simulink model "Comparacion_ANN"  (R2021a)
settings: Solver=VariableStepAuto  StartTime=0.0  StopTime=60  RelTol=1e-4
values from neighbouring files (symbols this model uses):
  selector = i    [Simulation.m]
undefined symbols (not defined in the file or in its folder): sigbuilder_block
libraries: spsDiodeLib x5, spsPVArrayLib x5, deeplib x4, simulink x4, spsCurrentMeasurementLib x1, spsControlledVoltageSourceLib x1, spsVoltageMeasurementLib x1, spspowerguiLib x1
settings Model: Creator=Guillermo  LastModifiedBy=Guillermo

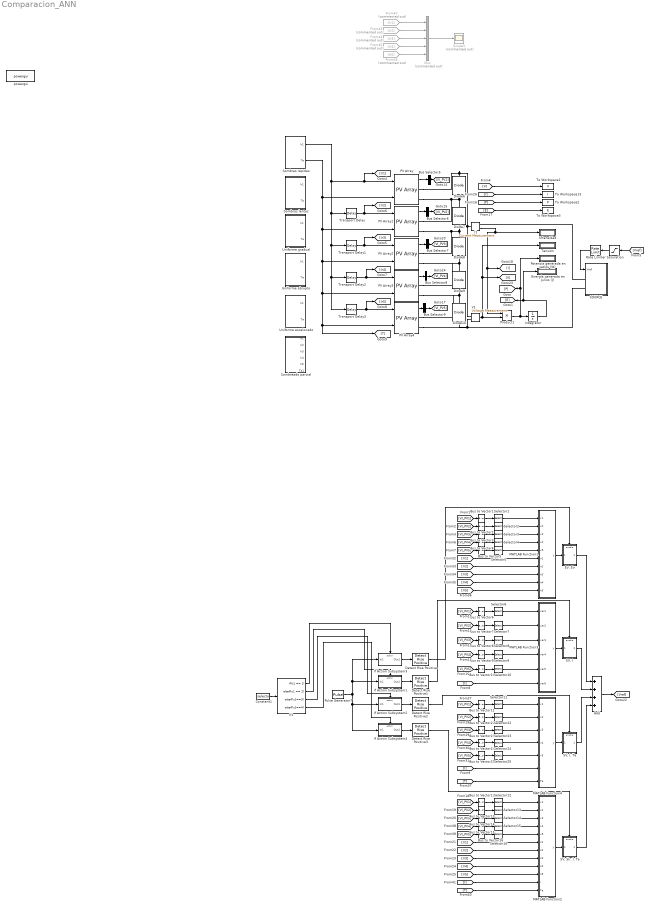
== system Comparacion_ANN ==
  "5V, 5Ir" : Subsystem
  "5V, 5Ir, I, Ta" : Subsystem
  "5V, I" : Subsystem
  "5V, I, Ta" : Subsystem
  Add : Sum  Inputs=++++
  Bus Selector{5..9} (5 alike) : BusSelector  OutputSignals=V_PV,I_PV  OutputAsBus=on
  Bus to Vector{1..16,22..25} (20 alike) : BusToVector
  Constant1 : Constant  Value=selector
  Detect Rise Positive{,1..3} (4 alike) : simulink/Logic and Bit Operations/Detect Rise Positive  vinit=0  OutDataTypeStr=boolean
  Diode{6..10} (5 alike) : spsDiodeLib/Diode  Ron=0.001  Lon=0  Vf=0.7  IC=0  UseSnubber=off  Rs=1e5*inf  Cs=inf  Measurements=off
  "Energía generada en Julios (J) " : Display
  From42 : From  Commented=on  GotoTag=Ir1
  From43 : From  Commented=on  GotoTag=Ir2
  From44 : From  Commented=on  GotoTag=Ir3
  From45 : From  Commented=on  GotoTag=Ir4
  From46 : From  Commented=on  GotoTag=Ir5
  I1 : spsCurrentMeasurementLib/Current Measurement  PhasorSimulation=off  OutputType=Complex  PSBequivalent=0
  If Action Subsystem1 : Subsystem  TreatAsAtomicUnit=on
  If Action Subsystem2 : Subsystem  TreatAsAtomicUnit=on
  If Action Subsystem3 : Subsystem  TreatAsAtomicUnit=on
  If Action Subsystem4 : Subsystem  TreatAsAtomicUnit=on
  If1 : If  IfExpression=u1 == 1  ElseIfExpressions=u1 == 2, u1==3, u1==4  ShowElse=off
  Integrator : Integrator
  Intensidad : Display
  MATLAB Function1 : MATLAB Function  TreatAsAtomicUnit=on
  MATLAB Function2 : MATLAB Function  TreatAsAtomicUnit=on
  MATLAB Function3 : MATLAB Function  TreatAsAtomicUnit=on
  MATLAB Function4 : MATLAB Function  TreatAsAtomicUnit=on
  Mux : Mux  Commented=on  Inputs=5
  PV Array{,1..4} (5 alike) : spsPVArrayLib/PV Array  Npar=1  Nser=1  PlotType=array @ 1000 W/m2 & specified temperatures  S_vec="[ 1000  500  100 ]"  Temp_C_vec="[ 45 25  ]"  ModuleName=SunPower SPR-305E-WHT-D  PlotWhenSelected=off  Pm=305.226  Ncell=96  Voc=64.2  Isc=5.96  Vm=54.7  Im=5.58  beta_Voc_pc=-0.2727  alpha_Isc_pc=0.061745  beta_Voc=-0.17507  alpha_Isc=0.00368  IL=5.9657  I0=6.3076e-12  nI=0.94489  Rsh=393.2054  Rs=0.37428  RobustModel=off  RobustCellTemperature=313.3991  BAL=on  Tc=1e-3  Tfilter=5e-5
  "Potencia generada en vatios (W) " : Display
  Product1 : Product
  Pulse Generator7 : DiscretePulseGenerator  PulseType=Time based  Period=1e-3  PulseWidth=20
      settings: AttributesFormatString=Period: %<period>\nDuty cycle: %<pulsewidth>%
  Rate Limiter : RateLimiter  RisingSlewLimit=100000  FallingSlewLimit=-100000  SampleTimeMode=inherited  InitialCondition=150
  SOURCE : Subsystem
  Saturation : Saturate  UpperLimit=290  LowerLimit=40
  Scope3 : Scope  Commented=on
  Selector{1..16,22..25} (20 alike) : Selector  InputPortWidth=2  IndexOptions=Index vector (dialog)  Indices=[1]  OutputSizes=1
  Sombras lentas : Subsystem  Tag=STV Subsys  LoadFcn=sigbuilder_block('load');  StartFcn=sigbuilder_block('start');  StopFcn=sigbuilder_block('stop');  ClipboardFcn=sigbuilder_block('clipboard');  mask(Sigbuilder block){tuvar=[0:10]}
      mask help: Simulink:masks:SigbuilderBlock_MD
      mask init:
      | if ~strcmp(get_param(bdroot(gcbh),'SimulationStatus'),'stopped') tuvar = sigbuilder_block('maskInit'); end
      settings: CopyFcn=sigbuilder_block('copy');  DeleteFcn=sigbuilder_block('delete');  ModelCloseFcn=sigbuilder_block('modelClose');  PreSaveFcn=sigbuilder_block('preSave');  PauseFcn=sigbuilder_block('pause');  ContinueFcn=sigbuilder_block('continue');  NameChangeFcn=sigbuilder_block('namechange');  OpenFcn=sigbuilder_block('open',[6 30 1908 951.75 ]);  CloseFcn=sigbuilder_block('close');
      mask Display: plot(0, 0, 100, 100,[2, 2, 32, 32, 2], [68, 8, 8, 68, 68],[32, 2], [38, 38], [32, 19, 2],[53, 60, 44], [32, 17, 17, 2],[16, 16, 31, 31]);txt = getActiveGroup(gcbh);text(2, 100, txt,'verticalAlignment', 'top');
  Sombras rápidas : Subsystem  Tag=STV Subsys  LoadFcn=sigbuilder_block('load');  StartFcn=sigbuilder_block('start');  StopFcn=sigbuilder_block('stop');  ClipboardFcn=sigbuilder_block('clipboard');  mask(Sigbuilder block){tuvar=[0:10]}
      mask help: Simulink:masks:SigbuilderBlock_MD
      mask init:
      | if ~strcmp(get_param(bdroot(gcbh),'SimulationStatus'),'stopped') tuvar = sigbuilder_block('maskInit'); end
      settings: CopyFcn=sigbuilder_block('copy');  DeleteFcn=sigbuilder_block('delete');  ModelCloseFcn=sigbuilder_block('modelClose');  PreSaveFcn=sigbuilder_block('preSave');  PauseFcn=sigbuilder_block('pause');  ContinueFcn=sigbuilder_block('continue');  NameChangeFcn=sigbuilder_block('namechange');  OpenFcn=sigbuilder_block('open',[6 30 1908 951.75 ]);  CloseFcn=sigbuilder_block('close');
      mask Display: plot(0, 0, 100, 100,[2, 2, 32, 32, 2], [68, 8, 8, 68, 68],[32, 2], [38, 38], [32, 19, 2],[53, 60, 44], [32, 17, 17, 2],[16, 16, 31, 31]);txt = getActiveGroup(gcbh);text(2, 100, txt,'verticalAlignment', 'top');
  Sombreado parcial : Subsystem  Tag=STV Subsys  LoadFcn=sigbuilder_block('load');  StartFcn=sigbuilder_block('start');  StopFcn=sigbuilder_block('stop');  ClipboardFcn=sigbuilder_block('clipboard');  mask(Sigbuilder block){tuvar=[0:10]}
      mask help: Simulink:masks:SigbuilderBlock_MD
      mask init:
      | if ~strcmp(get_param(bdroot(gcbh),'SimulationStatus'),'stopped') tuvar = sigbuilder_block('maskInit'); end
      settings: CopyFcn=sigbuilder_block('copy');  DeleteFcn=sigbuilder_block('delete');  ModelCloseFcn=sigbuilder_block('modelClose');  PreSaveFcn=sigbuilder_block('preSave');  PauseFcn=sigbuilder_block('pause');  ContinueFcn=sigbuilder_block('continue');  NameChangeFcn=sigbuilder_block('namechange');  OpenFcn=sigbuilder_block('open',[6 30 1908 951.75 ]);  CloseFcn=sigbuilder_block('close');
      mask Display: plot(0, 0, 100, 100,[2, 2, 32, 32, 2], [68, 8, 8, 68, 68],[32, 2], [38, 38], [32, 19, 2],[53, 60, 44], [32, 17, 17, 2],[16, 16, 31, 31]);txt = getActiveGroup(gcbh);text(2, 100, txt,'verticalAlignment', 'top');
  Tensión : Display
  To Workspace1 : ToWorkspace  VariableName=V  SampleTime=1e-3
  To Workspace13 : ToWorkspace  VariableName=I  SampleTime=1e-3
  To Workspace2 : ToWorkspace  VariableName=P  SampleTime=1e-3
  To Workspace3 : ToWorkspace  VariableName=E  SampleTime=1e-3
  Transport Delay : TransportDelay  DelayTime=0.1  InitialOutput=1000
  Transport Delay1 : TransportDelay  DelayTime=0.2  InitialOutput=1000
  Transport Delay2 : TransportDelay  DelayTime=0.3  InitialOutput=1000
  Transport Delay3 : TransportDelay  DelayTime=0.4  InitialOutput=1000
  Uniforme abrupto : Subsystem  Tag=STV Subsys  LoadFcn=sigbuilder_block('load');  StartFcn=sigbuilder_block('start');  StopFcn=sigbuilder_block('stop');  ClipboardFcn=sigbuilder_block('clipboard');  mask(Sigbuilder block){tuvar=[0:10]}
      mask help: Simulink:masks:SigbuilderBlock_MD
      mask init:
      | if ~strcmp(get_param(bdroot(gcbh),'SimulationStatus'),'stopped') tuvar = sigbuilder_block('maskInit'); end
      settings: CopyFcn=sigbuilder_block('copy');  DeleteFcn=sigbuilder_block('delete');  ModelCloseFcn=sigbuilder_block('modelClose');  PreSaveFcn=sigbuilder_block('preSave');  PauseFcn=sigbuilder_block('pause');  ContinueFcn=sigbuilder_block('continue');  NameChangeFcn=sigbuilder_block('namechange');  OpenFcn=sigbuilder_block('open',[6 30 1908 951.75 ]);  CloseFcn=sigbuilder_block('close');
      mask Display: plot(0, 0, 100, 100,[2, 2, 32, 32, 2], [68, 8, 8, 68, 68],[32, 2], [38, 38], [32, 19, 2],[53, 60, 44], [32, 17, 17, 2],[16, 16, 31, 31]);txt = getActiveGroup(gcbh);text(2, 100, txt,'verticalAlignment', 'top');
  Uniforme escalonado : Subsystem  Tag=STV Subsys  LoadFcn=sigbuilder_block('load');  StartFcn=sigbuilder_block('start');  StopFcn=sigbuilder_block('stop');  ClipboardFcn=sigbuilder_block('clipboard');  mask(Sigbuilder block){tuvar=[0:10]}
      mask help: Simulink:masks:SigbuilderBlock_MD
      mask init:
      | if ~strcmp(get_param(bdroot(gcbh),'SimulationStatus'),'stopped') tuvar = sigbuilder_block('maskInit'); end
      settings: CopyFcn=sigbuilder_block('copy');  DeleteFcn=sigbuilder_block('delete');  ModelCloseFcn=sigbuilder_block('modelClose');  PreSaveFcn=sigbuilder_block('preSave');  PauseFcn=sigbuilder_block('pause');  ContinueFcn=sigbuilder_block('continue');  NameChangeFcn=sigbuilder_block('namechange');  OpenFcn=sigbuilder_block('open',[6 30 1908 951.75 ]);  CloseFcn=sigbuilder_block('close');
      mask Display: plot(0, 0, 100, 100,[2, 2, 32, 32, 2], [68, 8, 8, 68, 68],[32, 2], [38, 38], [32, 19, 2],[53, 60, 44], [32, 17, 17, 2],[16, 16, 31, 31]);txt = getActiveGroup(gcbh);text(2, 100, txt,'verticalAlignment', 'top');
  Uniforme gradual : Subsystem  Tag=STV Subsys  LoadFcn=sigbuilder_block('load');  StartFcn=sigbuilder_block('start');  StopFcn=sigbuilder_block('stop');  ClipboardFcn=sigbuilder_block('clipboard');  mask(Sigbuilder block){tuvar=[0:10]}
      mask help: Simulink:masks:SigbuilderBlock_MD
      mask init:
      | if ~strcmp(get_param(bdroot(gcbh),'SimulationStatus'),'stopped') tuvar = sigbuilder_block('maskInit'); end
      settings: CopyFcn=sigbuilder_block('copy');  DeleteFcn=sigbuilder_block('delete');  ModelCloseFcn=sigbuilder_block('modelClose');  PreSaveFcn=sigbuilder_block('preSave');  PauseFcn=sigbuilder_block('pause');  ContinueFcn=sigbuilder_block('continue');  NameChangeFcn=sigbuilder_block('namechange');  OpenFcn=sigbuilder_block('open',[6 30 1908 951.75 ]);  CloseFcn=sigbuilder_block('close');
      mask Display: plot(0, 0, 100, 100,[2, 2, 32, 32, 2], [68, 8, 8, 68, 68],[32, 2], [38, 38], [32, 19, 2],[53, 60, 44], [32, 17, 17, 2],[16, 16, 31, 31]);txt = getActiveGroup(gcbh);text(2, 100, txt,'verticalAlignment', 'top');
  V1 : spsVoltageMeasurementLib/Voltage Measurement  PhasorSimulation=off  OutputType=Complex  PSBequivalent=0
  powergui : spspowerguiLib/powergui  Priority=1  SimulationMode=Continuous  SampleTime=1e-7  frequency=60  Iterations=50  frequencyindice=0  Pbase=100e6  ErrMax=1e-4  UnitsV=kV  UnitsW=MW  buscounter=0  FunctionMessages=off  echomessages=off  EnableUseOfTLC=off  CurrentSourceSwitches=off  DisableSnubberDevices=on  DisableRonSwitches=off  DisableVfSwitches=off  DisplayEquations=off  AutomaticDiscreteSolvers=off  SolverType=Tustin/Backward Euler (TBE)  Interpol=off  ExternalGateDelay=off  methode=off  Ts=0  x0status=blocks  SPID=off  SwTol=0  HookPort=off  NonlinearTolerance=1e-4  nMaxIteration=100  ContinueOnMaxIteration=off  RestoreLinks=warning  ResistiveCurrentMeasurement=off  Frange=[0:2:500]  Ylog=off  Xlog=on  ShowGrid=off  save=off  variable=ZData  structure=0  ZoomFFT=on  StartTime=0.0  cycles=1  DisplayStyle=1  fundamental=60  FreqAxis=off  MaxFrequency=1000  frequencyindicesteady=1  RmsSteady=1  display=off
  wires:
  Bus Selector9/1 -> [VI_PV5]
  Bus Selector7/1 -> [VI_PV3]
  [I] -> MATLAB Function3/6(var6)
  Bus Selector5/1 -> [VI_PV1]
  [T] -> MATLAB Function4/7(Ta)
  [I] -> MATLAB Function4/6(i)
  V1/1 -> Tensión/1, [V], Product1/2
  PV Array2/1 -> Bus Selector7/1
  [I] -> To Workspace13/1
  Bus Selector8/1 -> [VI_PV4]
  [V] -> To Workspace1/1
  PV Array3/1 -> Bus Selector8/1
  Bus Selector6/1 -> [VI_PV2]
  PV Array/1 -> Bus Selector5/1
  PV Array1/1 -> Bus Selector6/1
  I1/1 -> Product1/1, [I], Intensidad/1
  PV Array4/1 -> Bus Selector9/1
  Integrator/1 -> "Energía generada en Julios (J) "/1, [E]
  Product1/1 -> [P], "Potencia generada en vatios (W) "/1, Integrator/1
  Bus to Vector4/1 -> Selector4/1
  Bus to Vector2/1 -> Selector2/1
  [VI_PV1] -> Bus to Vector1/1
  Bus to Vector3/1 -> Selector3/1
  [VI_PV3] -> Bus to Vector3/1
  Bus to Vector1/1 -> Selector1/1
  Bus to Vector5/1 -> Selector5/1
  Selector1/1 -> MATLAB Function1/1(v1)
  Selector5/1 -> MATLAB Function1/5(v5)
  Selector4/1 -> MATLAB Function1/4(v4)
  [VI_PV4] -> Bus to Vector4/1
  [VI_PV5] -> Bus to Vector5/1
  Selector3/1 -> MATLAB Function1/3(v3)
  [VI_PV2] -> Bus to Vector2/1
  Selector2/1 -> MATLAB Function1/2(v2)
  Bus to Vector9/1 -> Selector9/1
  Bus to Vector7/1 -> Selector7/1
  [VI_PV1] -> Bus to Vector6/1
  Bus to Vector8/1 -> Selector8/1
  [VI_PV3] -> Bus to Vector8/1
  Bus to Vector6/1 -> Selector6/1
  Bus to Vector10/1 -> Selector10/1
  Selector6/1 -> MATLAB Function3/1(var1)
  Selector10/1 -> MATLAB Function3/5(var5)
  Selector9/1 -> MATLAB Function3/4(var4)
  [VI_PV4] -> Bus to Vector9/1
  [VI_PV5] -> Bus to Vector10/1
  Selector8/1 -> MATLAB Function3/3(var3)
  [VI_PV2] -> Bus to Vector7/1
  Selector7/1 -> MATLAB Function3/2(var2)
  Bus to Vector24/1 -> Selector24/1
  Bus to Vector22/1 -> Selector22/1
  [VI_PV1] -> Bus to Vector11/1
  Bus to Vector23/1 -> Selector23/1
  [VI_PV3] -> Bus to Vector23/1
  Bus to Vector11/1 -> Selector11/1
  Bus to Vector25/1 -> Selector25/1
  Selector11/1 -> MATLAB Function4/1(v1)
  Selector25/1 -> MATLAB Function4/5(v5)
  Selector24/1 -> MATLAB Function4/4(v4)
  [VI_PV4] -> Bus to Vector24/1
  [VI_PV5] -> Bus to Vector25/1
  Selector23/1 -> MATLAB Function4/3(v3)
  [VI_PV2] -> Bus to Vector22/1
  Selector22/1 -> MATLAB Function4/2(v2)
  [Ir5] -> MATLAB Function1/10(ir5)
  [Ir4] -> MATLAB Function1/9(ir4)
  [Ir3] -> MATLAB Function1/8(ir3)
  [Ir2] -> MATLAB Function1/7(ir2)
  [Ir1] -> MATLAB Function1/6(ir1)
  [P] -> To Workspace2/1
  [E] -> To Workspace3/1
  "5V, 5Ir"/1(Out1) -> Add/1
  MATLAB Function1/1(y) -> "5V, 5Ir"/1(In1)
  MATLAB Function3/1(y) -> "5V, I"/1(In1)
  "5V, I"/1(Out1) -> Add/2
  MATLAB Function4/1(y) -> "5V, I, Ta"/1(In1)
  "5V, I, Ta"/1(Out1) -> Add/3
  "5V, 5Ir, I, Ta"/1(Out1) -> Add/4
  MATLAB Function2/1(y) -> "5V, 5Ir, I, Ta"/1(In1)
  Selector15/1 -> MATLAB Function2/4(v4)
  [Ir1] -> MATLAB Function2/6(ir1)
  [Ir2] -> MATLAB Function2/7(ir2)
  [Ir3] -> MATLAB Function2/8(ir3)
  Bus to Vector16/1 -> Selector16/1
  [Ir4] -> MATLAB Function2/9(ir4)
  [Ir5] -> MATLAB Function2/10(ir5)
  Bus to Vector13/1 -> Selector13/1
  Bus to Vector12/1 -> Selector12/1
  Bus to Vector15/1 -> Selector15/1
  Selector14/1 -> MATLAB Function2/3(v3)
  [VI_PV5] -> Bus to Vector16/1
  Selector16/1 -> MATLAB Function2/5(v5)
  [VI_PV2] -> Bus to Vector13/1
  [VI_PV1] -> Bus to Vector12/1
  Bus to Vector14/1 -> Selector14/1
  Selector12/1 -> MATLAB Function2/1(v1)
  Selector13/1 -> MATLAB Function2/2(v2)
  [VI_PV3] -> Bus to Vector14/1
  [VI_PV4] -> Bus to Vector15/1
  [T] -> MATLAB Function2/12(Ta)
  [I] -> MATLAB Function2/11(i)
  From45/1 -> Mux/4
  From46/1 -> Mux/5
  From42/1 -> Mux/1
  From43/1 -> Mux/2
  From44/1 -> Mux/3
  Mux/1 -> Scope3/1
  Saturation/1 -> Rate Limiter/1
  Constant1/1 -> If1/1
  If Action Subsystem1/1(Out1) -> Detect Rise Positive1/1
  If Action Subsystem2/1(Out1) -> Detect Rise Positive2/1
  If Action Subsystem4/1(Out1) -> Detect Rise Positive3/1
  If1/2 -> If Action Subsystem1/Action
  Pulse Generator7/1 -> If Action Subsystem3/1(In1), If Action Subsystem1/1(In1), If Action Subsystem4/1(In1), If Action Subsystem2/1(In1)
  If1/1 -> If Action Subsystem3/Action
  If1/3 -> If Action Subsystem2/Action
  If1/4 -> If Action Subsystem4/Action
  Detect Rise Positive1/1 -> "5V, I"/Enable
  Detect Rise Positive/1 -> "5V, 5Ir"/Enable
  Detect Rise Positive2/1 -> "5V, I, Ta"/Enable
  Detect Rise Positive3/1 -> "5V, 5Ir, I, Ta"/Enable
  Add/1 -> [Vref]
  Transport Delay/1 -> [Ir2], PV Array1/1
  Transport Delay1/1 -> PV Array2/1, [Ir3]
  Transport Delay2/1 -> [Ir4], PV Array3/1
  Transport Delay3/1 -> [Ir5], PV Array4/1
  Sombras rápidas/1(Ir1) -> Transport Delay3/1, Transport Delay2/1, Transport Delay1/1, Transport Delay/1, [Ir1], PV Array/1
  Sombras rápidas/2(Ta) -> PV Array/2, PV Array1/2, PV Array2/2, PV Array3/2, PV Array4/2, [T]
  [Vref] -> Saturation/1
  Rate Limiter/1 -> SOURCE/1(Vref)
  If Action Subsystem3/1(Out1) -> Detect Rise Positive/1
  connections:
  PV Array4/RConn1 -- PV Array3/RConn2 -- Diode10/RConn1 -- Diode9/LConn1
  Diode7/RConn1 -- Diode6/LConn1 -- PV Array1/RConn1 -- PV Array/RConn2
  SOURCE/LConn2 -- PV Array4/RConn2 -- Diode10/LConn1 -- V1/LConn2
  Diode8/RConn1 -- Diode7/LConn1 -- PV Array2/RConn1 -- PV Array1/RConn2
  Diode6/RConn1 -- I1/LConn1 -- V1/LConn1 -- PV Array/RConn1
  PV Array3/RConn1 -- PV Array2/RConn2 -- Diode9/RConn1 -- Diode8/LConn1
  SOURCE/LConn1 -- I1/RConn1

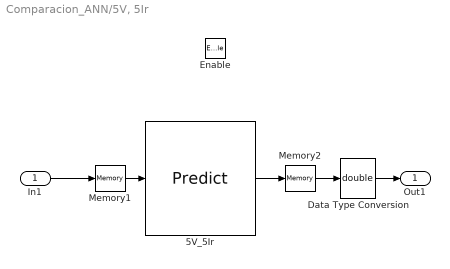
== system Comparacion_ANN/5V, 5Ir ==
  In1 : Inport
  Enable : EnablePort
  5V_5Ir : deeplib/Predict  Network=Network from MAT-file  NetworkFunction=squeezenet  NetworkFilePath=D:\Guillermo\Documentos\Universidad\TFG_E\MATLAB_FINAL\Comparacion_modelos_ANN\modelos_matlab\3_layers\5V_5Ir.mat  MiniBatchSize=256  InputDataFormats={ '', '' }  Predictions=on  Activations={}  ForceInterpretedSim=off  EnableDLNetwork=off
      settings: SourceProductBaseCode=NN
  Data Type Conversion : DataTypeConversion  OutDataTypeStr=double
  Memory1 : Memory
  Memory2 : Memory
  Out1 : Outport
  wires:
  Memory1/1 -> 5V_5Ir/1
  5V_5Ir/1 -> Memory2/1
  Memory2/1 -> Data Type Conversion/1
  In1/1 -> Memory1/1
  Data Type Conversion/1 -> Out1/1

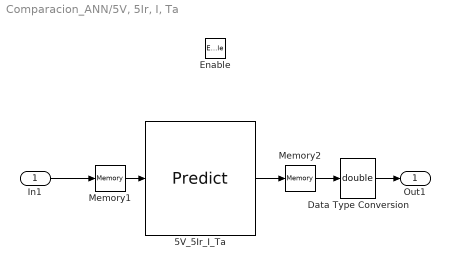
== system Comparacion_ANN/5V, 5Ir, I, Ta ==
  In1 : Inport
  Enable : EnablePort
  5V_5Ir_I_Ta : deeplib/Predict  Network=Network from MAT-file  NetworkFunction=squeezenet  NetworkFilePath=D:\Guillermo\Documentos\Universidad\TFG_E\MATLAB_FINAL\Comparacion_modelos_ANN\modelos_matlab\3_layers\5V_5Ir_I_Ta.mat  MiniBatchSize=256  InputDataFormats={ '', '' }  Predictions=on  Activations={}  ForceInterpretedSim=off  EnableDLNetwork=off
      settings: SourceProductBaseCode=NN
  Data Type Conversion : DataTypeConversion  OutDataTypeStr=double
  Memory1 : Memory
  Memory2 : Memory
  Out1 : Outport
  wires:
  Memory1/1 -> 5V_5Ir_I_Ta/1
  5V_5Ir_I_Ta/1 -> Memory2/1
  Memory2/1 -> Data Type Conversion/1
  In1/1 -> Memory1/1
  Data Type Conversion/1 -> Out1/1

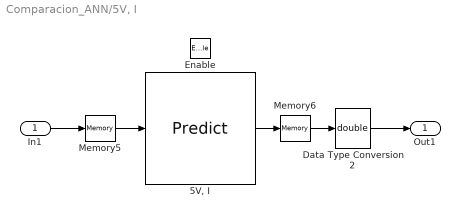
== system Comparacion_ANN/5V, I ==
  In1 : Inport
  Enable : EnablePort
  "5V, I" : deeplib/Predict  Network=Network from MAT-file  NetworkFunction=squeezenet  NetworkFilePath=D:\Guillermo\Documentos\Universidad\TFG_E\MATLAB_FINAL\Comparacion_modelos_ANN\modelos_matlab\3_layers\5V_I.mat  MiniBatchSize=256  InputDataFormats={ '', '' }  Predictions=on  Activations={}  ForceInterpretedSim=off  EnableDLNetwork=off
      settings: SourceProductBaseCode=NN
  Data Type Conversion2 : DataTypeConversion  OutDataTypeStr=double
  Memory5 : Memory
  Memory6 : Memory
  Out1 : Outport
  wires:
  Memory5/1 -> "5V, I"/1
  Memory6/1 -> Data Type Conversion2/1
  Data Type Conversion2/1 -> Out1/1
  "5V, I"/1 -> Memory6/1
  In1/1 -> Memory5/1

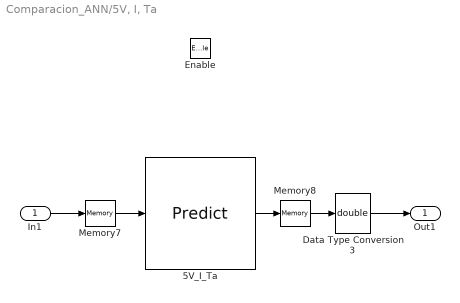
== system Comparacion_ANN/5V, I, Ta ==
  In1 : Inport
  Enable : EnablePort
  5V_I_Ta : deeplib/Predict  Network=Network from MAT-file  NetworkFunction=squeezenet  NetworkFilePath=D:\Guillermo\Documentos\Universidad\TFG_E\MATLAB_FINAL\Comparacion_modelos_ANN\modelos_matlab\3_layers\5V_I_Ta.mat  MiniBatchSize=256  InputDataFormats={ '', '' }  Predictions=on  Activations={}  ForceInterpretedSim=off  EnableDLNetwork=off
      settings: SourceProductBaseCode=NN
  Data Type Conversion3 : DataTypeConversion  OutDataTypeStr=double
  Memory7 : Memory
  Memory8 : Memory
  Out1 : Outport
  wires:
  Data Type Conversion3/1 -> Out1/1
  Memory7/1 -> 5V_I_Ta/1
  5V_I_Ta/1 -> Memory8/1
  Memory8/1 -> Data Type Conversion3/1
  In1/1 -> Memory7/1

== system Comparacion_ANN/If Action Subsystem1 ==
  In1 : Inport
  Action Port : ActionPort  InitializeStates=reset  ActionPortLabel=elseif(u1 == 2)
  Out1 : Outport
  wires:
  In1/1 -> Out1/1

== system Comparacion_ANN/If Action Subsystem2 ==
  In1 : Inport
  Action Port : ActionPort  InitializeStates=reset  ActionPortLabel=elseif( u1==3)
  Out1 : Outport
  wires:
  In1/1 -> Out1/1

== system Comparacion_ANN/If Action Subsystem3 ==
  In1 : Inport
  Action Port : ActionPort  InitializeStates=reset  ActionPortLabel=if(u1 == 1)
  Out1 : Outport
  wires:
  In1/1 -> Out1/1

== system Comparacion_ANN/If Action Subsystem4 ==
  In1 : Inport
  Action Port : ActionPort  InitializeStates=reset  ActionPortLabel=elseif( u1==4)
  Out1 : Outport
  wires:
  In1/1 -> Out1/1

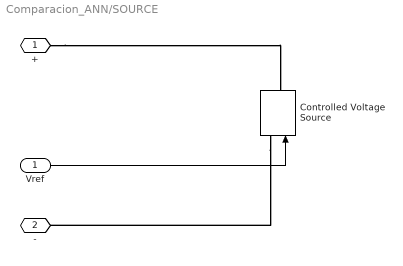
== system Comparacion_ANN/SOURCE ==
  Vref : Inport
  Controlled Voltage Source : spsControlledVoltageSourceLib/Controlled Voltage Source  Initialize=on  Source_Type=AC  Amplitude=0  Phase=0  Frequency=0  Measurements=None
  + : PMIOPort  Side=Left
  - : PMIOPort  Port=2  Side=Left
  wires:
  Vref/1 -> Controlled Voltage Source/1
  connections:
  Controlled Voltage Source/LConn1 -- -/RConn1
  +/RConn1 -- Controlled Voltage Source/RConn1

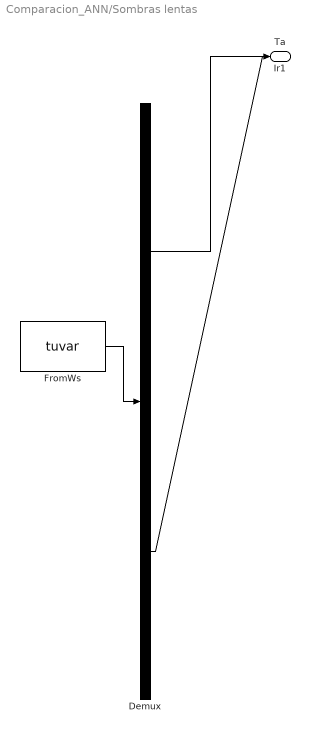
== system Comparacion_ANN/Sombras lentas ==
  Demux : Demux  Tag=STV Demux  Outputs=2
      settings: DisplayOption=none
  FromWs : FromWorkspace  Tag=STV FromWs  VariableName=tuvar
      SigBuilderData=|
      | common.afterFinalStr = 'Extrapolate'
      | common.sampleTime = 0
      | dataSet.timeRange = [0 60]
      | dataSet.name = 'Group 1'
      | sbobj.Groups.Name = 'Group 1'
      | sbobj.Groups.Signals(1).Name = 'Ir1'
      | sbobj.Groups.Signals(1).XData = [0 1 1.4 7 7.25 16.5 16.75 25.25 25.75 34.75 35 37 37.25 45 45.25 48 48.25 50 50.25 57 57.25 60]
      | sbobj.Groups.Signals(1).YData = [910 500 295 295 910 910 295 295 910 910 295 295 910 910 295 295 910 910 295 295 910 910]
      | sbobj.Groups.Signals(2).Name = 'Ta'
      | sbobj.Groups.Signals(2).XData = [0 60]
      | sbobj.Groups.Signals(2).YData = [22.6 22.6]
      | sbobj.Groups.TimeRange = [0 60]
  Ir1 : Outport  Tag=STV Outport
  Ta : Outport  Tag=STV Outport  Port=2
  wires:
  FromWs/1 -> Demux/1
  Demux/1 -> Ir1/1
  Demux/2 -> Ta/1

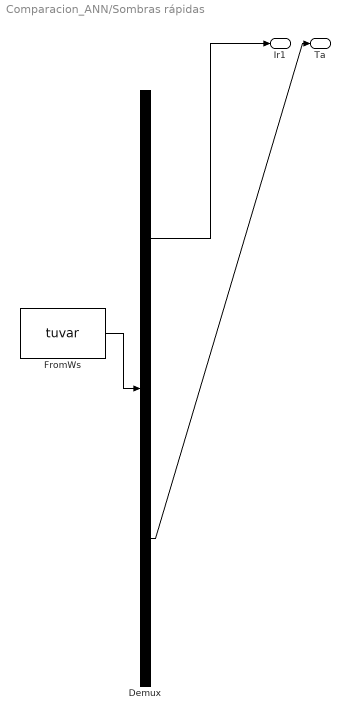
== system Comparacion_ANN/Sombras rápidas ==
  Demux : Demux  Tag=STV Demux  Outputs=2
      settings: DisplayOption=none
  FromWs : FromWorkspace  Tag=STV FromWs  VariableName=tuvar
      SigBuilderData=|
      | common.afterFinalStr = 'Extrapolate'
      | common.sampleTime = 0
      | dataSet.timeRange = [0 60]
      | dataSet.name = 'Group 1'
      | sbobj.Groups.Name = 'Group 1'
      | sbobj.Groups.Signals(1).Name = 'Ir1'
      | sbobj.Groups.Signals(1).XData = [0 1 1.4 7 7.25 10 10.25 10.5 12 12.25 16 16.25 16.5 16.75 18.95 19.5 20 21.05 24 24.5 25 25.25 25.75 29 32 32.25 34 34.25 34.5 34.75 35 37 37.25 41 41.25 41.5 41.75 42 45 45.25 48 48.25 50 50.25 53.75 54 54.25 57 57.25 60]
      | sbobj.Groups.Signals(1).YData = [910 500 295 295 910 910 295 295 295 910 910 295 910 295 295 910 295 910 910 290 910 295 910 910 910 295 295 910 295 910 295 295 910 910 295 910 295 910 910 295 295 910 910 295 295 910 295 295 910 910]
      | sbobj.Groups.Signals(2).Name = 'Ta'
      | sbobj.Groups.Signals(2).XData = [0 60]
      | sbobj.Groups.Signals(2).YData = [22.6 22.6]
      | sbobj.Groups.TimeRange = [0 60]
  Ir1 : Outport  Tag=STV Outport
  Ta : Outport  Tag=STV Outport  Port=2
  wires:
  FromWs/1 -> Demux/1
  Demux/1 -> Ir1/1
  Demux/2 -> Ta/1

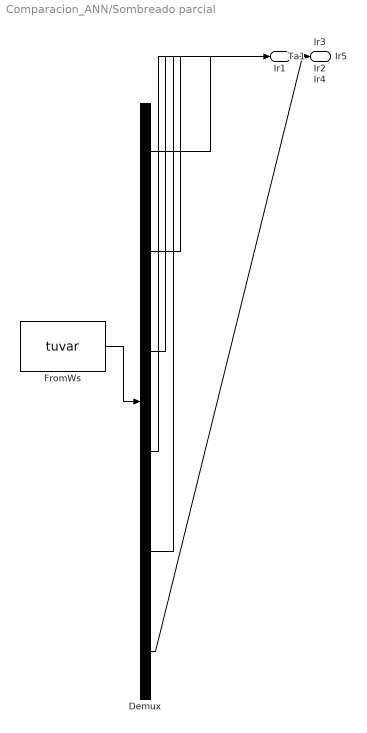
== system Comparacion_ANN/Sombreado parcial ==
  Demux : Demux  Tag=STV Demux  Outputs=6
      settings: DisplayOption=none
  FromWs : FromWorkspace  Tag=STV FromWs  VariableName=tuvar
      SigBuilderData=|
      | common.afterFinalStr = 'Extrapolate'
      | common.sampleTime = 0
      | dataSet.timeRange = [0 60]
      | dataSet.name = 'Group 1'
      | sbobj.Groups.Name = 'Group 1'
      | sbobj.Groups.Signals(1).Name = 'Ir1'
      | sbobj.Groups.Signals(1).XData = [0 30 30.25 60]
      | sbobj.Groups.Signals(1).YData = [900 900 300 300]
      | sbobj.Groups.Signals(2).Name = 'Ir2'
      | sbobj.Groups.Signals(2).XData = [0 30 30.25 60]
      | sbobj.Groups.Signals(2).YData = [909 900 300 295]
      | sbobj.Groups.Signals(3).Name = 'Ir3'
      | sbobj.Groups.Signals(3).XData = [0 30 30.25 60]
      | sbobj.Groups.Signals(3).YData = [900 900 300 300]
      | sbobj.Groups.Signals(4).Name = 'Ir4'
      | sbobj.Groups.Signals(4).XData = [0 30 30.25 60]
      | sbobj.Groups.Signals(4).YData = [300 300 900 900]
      | sbobj.Groups.Signals(5).Name = 'Ir5'
      | sbobj.Groups.Signals(5).XData = [0 30 30.25 60]
      | sbobj.Groups.Signals(5).YData = [300 300 900 900]
      | sbobj.Groups.Signals(6).Name = 'Ta1'
      | sbobj.Groups.Signals(6).XData = [0 60]
      | sbobj.Groups.Signals(6).YData = [22.6 22.6]
      | sbobj.Groups.TimeRange = [0 60]
  Ir1 : Outport  Tag=STV Outport
  Ir2 : Outport  Tag=STV Outport  Port=2
  Ir3 : Outport  Tag=STV Outport  Port=3
  Ir4 : Outport  Tag=STV Outport  Port=4
  Ir5 : Outport  Tag=STV Outport  Port=5
  Ta1 : Outport  Tag=STV Outport  Port=6
  wires:
  FromWs/1 -> Demux/1
  Demux/1 -> Ir1/1
  Demux/2 -> Ir2/1
  Demux/3 -> Ir3/1
  Demux/4 -> Ir4/1
  Demux/5 -> Ir5/1
  Demux/6 -> Ta1/1

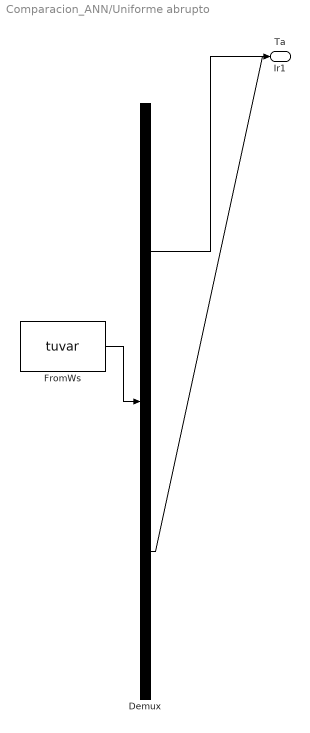
== system Comparacion_ANN/Uniforme abrupto ==
  Demux : Demux  Tag=STV Demux  Outputs=2
      settings: DisplayOption=none
  FromWs : FromWorkspace  Tag=STV FromWs  VariableName=tuvar
      SigBuilderData=|
      | common.afterFinalStr = 'Extrapolate'
      | common.sampleTime = 0
      | dataSet.timeRange = [0 60]
      | dataSet.name = 'Group 1'
      | sbobj.Groups.Name = 'Group 1'
      | sbobj.Groups.Signals(1).Name = 'Ir1'
      | sbobj.Groups.Signals(1).XData = [0 30 30.25 60]
      | sbobj.Groups.Signals(1).YData = [1000 1000 200 200]
      | sbobj.Groups.Signals(2).Name = 'Ta'
      | sbobj.Groups.Signals(2).XData = [0 60]
      | sbobj.Groups.Signals(2).YData = [22.6 22.6]
      | sbobj.Groups.TimeRange = [0 60]
  Ir1 : Outport  Tag=STV Outport
  Ta : Outport  Tag=STV Outport  Port=2
  wires:
  FromWs/1 -> Demux/1
  Demux/1 -> Ir1/1
  Demux/2 -> Ta/1

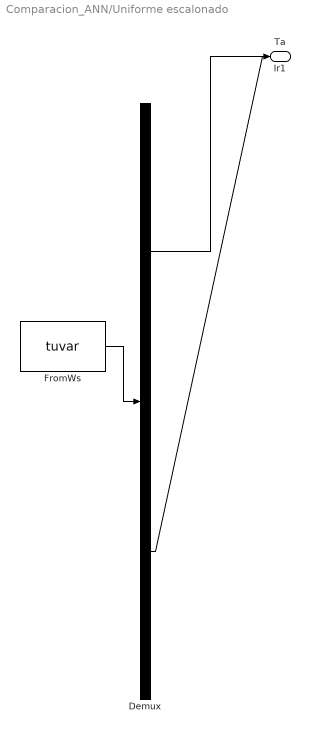
== system Comparacion_ANN/Uniforme escalonado ==
  Demux : Demux  Tag=STV Demux  Outputs=2
      settings: DisplayOption=none
  FromWs : FromWorkspace  Tag=STV FromWs  VariableName=tuvar
      SigBuilderData=|
      | common.afterFinalStr = 'Extrapolate'
      | common.sampleTime = 0
      | dataSet.timeRange = [0 60]
      | dataSet.name = 'Group 1'
      | sbobj.Groups.Name = 'Group 1'
      | sbobj.Groups.Signals(1).Name = 'Ir1'
      | sbobj.Groups.Signals(1).XData = [0 15 15.25 30 30.25 45 45.25 60]
      | sbobj.Groups.Signals(1).YData = [1000 1000 800 800 600 600 400 400]
      | sbobj.Groups.Signals(2).Name = 'Ta'
      | sbobj.Groups.Signals(2).XData = [0 60]
      | sbobj.Groups.Signals(2).YData = [22.6 22.6]
      | sbobj.Groups.TimeRange = [0 60]
  Ir1 : Outport  Tag=STV Outport
  Ta : Outport  Tag=STV Outport  Port=2
  wires:
  FromWs/1 -> Demux/1
  Demux/1 -> Ir1/1
  Demux/2 -> Ta/1

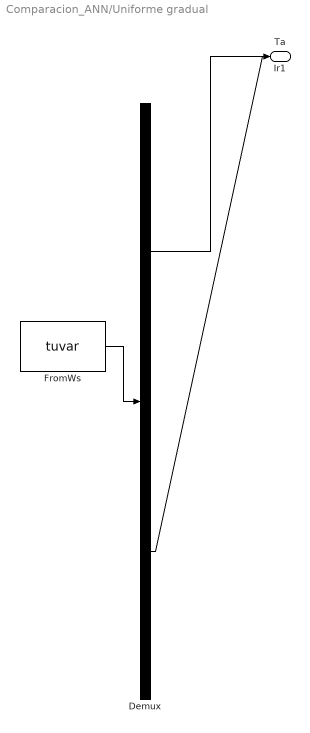
== system Comparacion_ANN/Uniforme gradual ==
  Demux : Demux  Tag=STV Demux  Outputs=2
      settings: DisplayOption=none
  FromWs : FromWorkspace  Tag=STV FromWs  VariableName=tuvar
      SigBuilderData=|
      | common.afterFinalStr = 'Extrapolate'
      | common.sampleTime = 0
      | dataSet.timeRange = [0 60]
      | dataSet.name = 'Group 1'
      | sbobj.Groups.Name = 'Group 1'
      | sbobj.Groups.Signals(1).Name = 'Ir1'
      | sbobj.Groups.Signals(1).XData = [0 60]
      | sbobj.Groups.Signals(1).YData = [1000 200]
      | sbobj.Groups.Signals(2).Name = 'Ta'
      | sbobj.Groups.Signals(2).XData = [0 60]
      | sbobj.Groups.Signals(2).YData = [22.6 22.6]
      | sbobj.Groups.TimeRange = [0 60]
  Ir1 : Outport  Tag=STV Outport
  Ta : Outport  Tag=STV Outport  Port=2
  wires:
  FromWs/1 -> Demux/1
  Demux/1 -> Ir1/1
  Demux/2 -> Ta/1

== matlab function Comparacion_ANN/MATLAB Function1 ==
  data: v1 input; y output; v2 input; v3 input; v4 input; v5 input; ir1 input; ir2 input; ir3 input; ir4 input; ir5 input
function y = fcn(v1,v2,v3,v4,v5,ir1,ir2,ir3,ir4,ir5)
y = double([v1,v2,v3,v4,v5,ir1,ir2,ir3,ir4,ir5]);
end

== matlab function Comparacion_ANN/MATLAB Function3 ==
  data: var1 input; y output; var2 input; var3 input; var4 input; var5 input; var6 input
% function y = fcn(v1,v2,v3,v4,v5,i)
% y = double([v1,v2,v3,v4,v5,i]);
% end

function y = fcn(var1,var2,var3,var4,var5,var6)
y = double([var1,var2,var3,var4,var5,var6]);
end

== matlab function Comparacion_ANN/MATLAB Function4 ==
  data: v1 input; y output; v2 input; v3 input; v4 input; v5 input; i input; Ta input
function y = fcn(v1,v2,v3,v4,v5,i,Ta)
y = double([v1,v2,v3,v4,v5,i,Ta]);
 
end

== matlab function Comparacion_ANN/MATLAB Function2 ==
  data: v1 input; y output; v2 input; v3 input; v4 input; v5 input; ir1 input; ir2 input; ir3 input; ir4 input; ir5 input; i input; Ta input
function y = fcn(v1,v2,v3,v4,v5,ir1,ir2,ir3,ir4,ir5,i,Ta)
y = double([v1,v2,v3,v4,v5,ir1,ir2,ir3,ir4,ir5,i,Ta]);
 
end
